simulink model "ReadWrite_1Motor"  (R2021a)
settings: Solver=VariableStepAuto  StartTime=0.0  StopTime=inf  RelTol=1e-3
undefined symbols (not defined in the file): motor_IDs, Ts
libraries: dxlSimLibrary x5
settings Model: EnablePacing=on  Creator=MSI PC  LastModifiedBy=PHUC

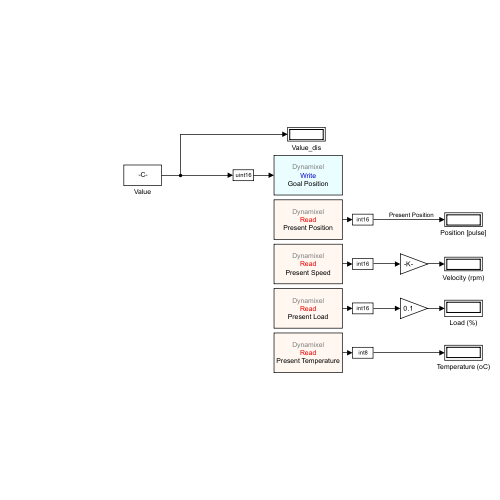
[thumbnail: Simulink's stored preview of the top-level diagram]
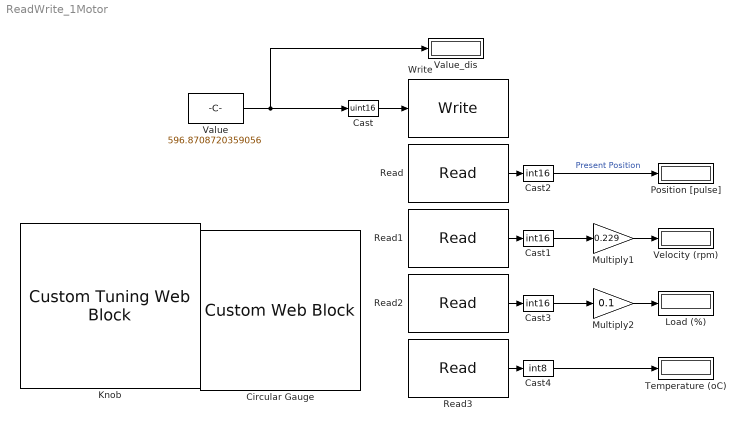
== system ReadWrite_1Motor ==
  Cast : DataTypeConversion  OutMin=0  OutMax=65535  OutDataTypeStr=uint16
  Cast1 : DataTypeConversion  OutDataTypeStr=int16
  Cast2 : DataTypeConversion  OutDataTypeStr=int16
  Cast3 : DataTypeConversion  OutDataTypeStr=int16
  Cast4 : DataTypeConversion  OutDataTypeStr=int8
  Circular Gauge : CustomWebBlock  LabelPosition=Hide  ShowInitialText=on  Configuration="{\"components\":[{\"name\":\"CircularScaleComponent\",\"settings\":{\"bounds\":{\"max\":1023,\"min\":0,\"tickInterval\":\"auto\"},\"direction\":\"cw\",\"flipLimits\":0,\"innerRadius\":0.75,\"internalTickHeightScaleFactor\":1,\"labelColor\":[0,0,0],\"labelFont\":{\"font\":\"Arial\",\"fontSize\":12},\"labelRadius\":0.6,\"labelTransparency\":1,\"minorTickHeightScaleFactor\":0.2,\"needleImage\":{\"size\":[200,50],\"src\":\"data:image\\/svg+xml;base64,PD94bWwgdmVyc2lvbj0iMS4wIiBlbmNvZGluZz0idXRmLTgiPz4KPCEtLSBHZW5lcmF0b3I6IEFkb2JlIElsbHVzdHJhdG9yIDI0LjEuMiwgU1ZHIEV4cG9ydCBQbHVnLUluIC4gU1ZHIFZlcnNpb246IDYuMDAgQnVpbGQgMCkgIC0tPgo8c3ZnIHZlcnNpb249IjEuMSIgaWQ9IkxheWVyXzEiIHhtbG5zPSJodHRwOi8vd3d3LnczLm9yZy8yMDAwL3N2ZyIgeG1sbnM6eGxpbms9Imh0dHA6Ly93d3cudzMub3JnLzE5OTkveGxpbmsiIHg9IjBweCIgeT0iMHB4IgoJIHZpZXdCb3g9IjAgMCAyMDAgNTAiIHN0eWxlPSJlbmFibGUtYmFja2dyb3VuZDpuZXcgMCAwIDIwMCA1MDsiIHhtbDpzcGFjZT0icHJlc2VydmUiPgo8c3R5bGUgdHlwZT0idGV4dC9jc3MiPgoJLnN0MHtmaWxsOiNFQzIxMjc7fQo8L3N0eWxlPgo8cGF0aCBjbGFzcz0ic3QwIiBkPSJNMTYyLjgsMTMuN0MxNjksNC40LDE4MS43LDEuOSwxOTEsOC4xczExLjgsMTguOSw1LjYsMjguMnMtMTguOSwxMS44LTI4LjIsNS42bDAsMAoJQzE1OS4xLDM1LjYsMTU2LjYsMjMsMTYyLjgsMTMuN0wxNjIuOCwxMy43eiBNMTY1LjgsMTUuOGMtNS4xLDcuNi0zLjEsMTcuOSw0LjYsMjNjNy42LDUuMSwxNy45LDMuMSwyMy00LjYKCWM1LjEtNy42LDMuMS0xNy45LTQuNi0yM2wwLDBDMTgxLjIsNi4yLDE3MC45LDguMiwxNjUuOCwxNS44eiIvPgo8cGF0aCBjbGFzcz0ic3QwIiBkPSJNMC40LDI1Ljl2LTMuM2wxNTktMi41Yy0wLjcsMi42LTAuNyw1LjIsMCw3LjhMMC40LDI1Ljl6Ii8+CjxjaXJjbGUgY2xhc3M9InN0MCIgY3g9IjE3OS42IiBjeT0iMjQiIHI9IjAuNyIvPgo8L3N2Zz4K\"},\"needleOffset\":[0.18464878250906522,0],\"needleOrientation\":-45,\"needleRotation\":180,\"needleSize\":{\"height\":0.11741692305346914,\"width\":0.46108337545091255},\"outerRadius\":0.9,\"position\":[0.0648561507936508,0.056299603174603176,0.8916790674603174,0.8787822420634921],\"referencePoint\":\"auto\",\"scaleAngle\":270,\"scaleAngleOffset\":135,\"scaleColors\":[],\"scaleColorsSize\":0.2,\"scaleDirection\":\"CW\",\"scalePosition\":[0,0,1,1],\"showLabels\":1,\"showMinorTicks\":1,\"showSpanLine\":1,\"showTicks\":1,\"tickColor\":[0,0,0],\"tickTransparency\":1,\"valueBarColor\":[0,114,189],\"valueBarPosition\":[0,0,1,1],\"valueBarSize\":0.2,\"valueBarTransparency\":0.3}},{\"name\":\"BackgroundImageComponent\",\"settings\":{\"image\":{\"size\":[0,0],\"src\":\"default\",\"srcOrientation\":[]},\"position\":[0,0,1,1],\"scaleMode\":\"0\"}},{\"name\":\"ForegroundImageComponent\",\"settings\":{\"image\":{\"size\":[0,0],\"src\":\"default\",\"srcOrientation\":[]},\"isForeground\":1,\"position\":[0,0,1,1],\"scaleMode\":\"0\"}}],\"settings\":{\"BindingType\":\"signal\",\"aspectRatio\":1.032258064516129,\"backgroundColor\":[0,0,0,\"1\"],\"backgroundOffset\":0.14,\"backgroundOpacity\":1,\"direction\":\"cw\",\"fixedAspectRatio\":\"on\",\"flipLimits\":0,\"orientation\":\"horizontal\",\"showBackgroundColor\":false,\"value\":0,\"version\":\"R2021a\"},\"type\":\"CircularGauge\"}"
  Knob : CustomTuningWebBlock  LabelPosition=Hide  ShowInitialText=on  Configuration="{\"components\":[{\"name\":\"CircularScaleComponent\",\"settings\":{\"bounds\":{\"max\":1023,\"min\":0,\"tickInterval\":100},\"direction\":\"cw\",\"flipLimits\":0,\"innerRadius\":0.6636618227670849,\"internalTickHeightScaleFactor\":1,\"labelColor\":[0,0,0],\"labelFont\":{\"font\":\"Arial\",\"fontSize\":12},\"labelRadius\":0.84,\"labelTransparency\":1,\"minorTickHeightScaleFactor\":0.2,\"needleImage\":{\"size\":[150,150],\"src\":\"data:image\\/svg+xml;base64,PD94bWwgdmVyc2lvbj0iMS4wIiBlbmNvZGluZz0idXRmLTgiPz4NCjwhLS0gR2VuZXJhdG9yOiBBZG9iZSBJbGx1c3RyYXRvciAyNS4yLjMsIFNWRyBFeHBvcnQgUGx1Zy1JbiAuIFNWRyBWZXJzaW9uOiA2LjAwIEJ1aWxkIDApICAtLT4NCjxzdmcgdmVyc2lvbj0iMS4xIiBpZD0iTGF5ZXJfMSIgeG1sbnM9Imh0dHA6Ly93d3cudzMub3JnLzIwMDAvc3ZnIiB4bWxuczp4bGluaz0iaHR0cDovL3d3dy53My5vcmcvMTk5OS94bGluayIgeD0iMHB4IiB5PSIwcHgiDQoJIHZpZXdCb3g9IjAgMCAxNTIgMTUyIiBzdHlsZT0iZW5hYmxl ...(+37472 chars)\"},\"needleOffset\":[0,0],\"needleOrientation\":-45,\"needleRotation\":90,\"needleSize\":{\"height\":0.44,\"width\":0.44},\"outerRadius\":0.5053386200069245,\"position\":[0.004878048780487805,0,1,1],\"referencePoint\":\"auto\",\"scaleAngle\":270,\"scaleAngleOffset\":135,\"scaleColors\":[],\"scaleColorsSize\":0.2,\"scaleDirection\":\"CW\",\"scalePosition\":[0,0,1,1],\"showLabels\":true,\"showMinorTicks\":1,\"showSpanLine\":true,\"showTicks\":1,\"tickColor\":[0,0,0],\"tickTransparency\":1,\"valueBarColor\":[0,114,189],\"valueBarPosition\":[0,0,1,1],\"valueBarSize\":0.2,\"valueBarTransparency\":0.3}},{\"name\":\"BackgroundImageComponent\",\"settings\":{\"image\":{\"size\":[0,0],\"src\":\"default\",\"srcOrientation\":[]},\"position\":[0,0,1,1],\"scaleMode\":\"0\"}},{\"name\":\"ForegroundImageComponent\",\"settings\":{\"image\":{\"size\":[0,0],\"src\":\"default\",\"srcOrientation\":[]},\"isForeground\":1,\"position\":[0,0,1,1],\"scaleMode\":\"0\"}}],\"settings\":{\"BindingType\":\"param\",\"aspectRatio\":1,\"backgroundColor\":[0,0,0],\"backgroundOffset\":1,\"backgroundOpacity\":1,\"direction\":\"cw\",\"fixedAspectRatio\":\"on\",\"flipLimits\":0,\"foregroundColor\":[252,252,196],\"orientation\":\"horizontal\",\"showBackgroundColor\":false,\"value\":0,\"version\":\"R2021a\"},\"type\":\"CircularGauge\"}"
  Load (%) : Display
  Multiply1 : Gain  Gain=0.229  OutDataTypeStr=double
  Multiply2 : Gain  Gain=0.1  OutDataTypeStr=double
  Position [pulse] : Display
  Read : dxlSimLibrary/Read  lib_name=lib_name  port_num=port_num  protocol_version=protocol_version  ids=motor_IDs(1)  models=motor_models  select=Present Position  Ts=Ts
  Read1 : dxlSimLibrary/Read  lib_name=lib_name  port_num=port_num  protocol_version=protocol_version  ids=motor_IDs(1)  models=motor_models  select=Present Speed  Ts=Ts
  Read2 : dxlSimLibrary/Read  lib_name=lib_name  port_num=port_num  protocol_version=protocol_version  ids=motor_IDs(1)  models=motor_models  select=Present Load  Ts=Ts
  Read3 : dxlSimLibrary/Read  lib_name=lib_name  port_num=port_num  protocol_version=protocol_version  ids=motor_IDs(1)  models=motor_models  select=Present Temperature  Ts=Ts
  Temperature (oC) : Display
  Value : Constant  Value=596.8708720359056  OutDataTypeStr=int32
  Value_dis : Display
  Velocity (rpm) : Display
  Write : dxlSimLibrary/Write  lib_name=lib_name  port_num=port_num  protocol_version=protocol_version  ids=motor_IDs(1)  models=motor_models  select=Goal Position  Ts=Ts
  wires:
  Cast/1 -> Write/1
  Value/1 -> Cast/1, Value_dis/1
  Read/1 -> Cast2/1
  Cast2/1 -> Position [pulse]/1  "Present Position"
  Read3/1 -> Cast4/1
  Read2/1 -> Cast3/1
  Read1/1 -> Cast1/1
  Cast1/1 -> Multiply1/1
  Multiply1/1 -> Velocity (rpm)/1
  Cast3/1 -> Multiply2/1
  Cast4/1 -> Temperature (oC)/1
  Multiply2/1 -> Load (%)/1
